simulink model "sampleModel1754"  (R2023a)
settings: Solver=VariableStepAuto  StartTime=0.0  StopTime=10.0  RelTol=1e-3
libraries: hdlsllib x5, simulink x1
settings Model: Creator=user1  LastModifiedBy=user1

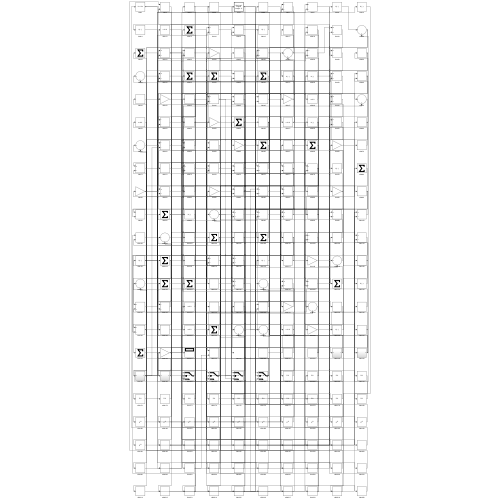
[thumbnail: Simulink's stored preview of the top-level diagram]
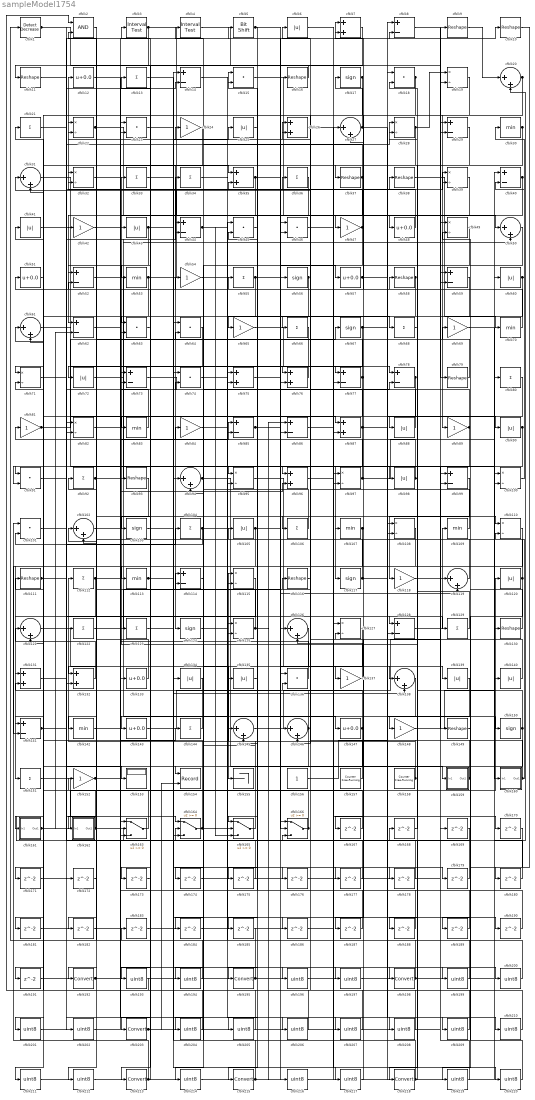
== system sampleModel1754 ==
  cfblk1 : simulink/Logic and Bit Operations/Detect Decrease  vinit=0.0  OutDataTypeStr=boolean
      settings: LibrarySourceBlock=|
      | hdlsllib/Logic and Bit
      | Operations/Detect
      | Decrease
  cfblk{9..11,16,37..38,58,79,93,111,116,130,149} (13 alike) : Reshape
  cfblk{19,22,28,32,39,49,71,82,95,97,100,108,110,115,125,127} (16 alike) : Product  Inputs=*/  RndMeth=Zero  SaturateOnIntegerOverflow=on
  cfblk{15,18,23,45..46,63..64,74,91,101,136} (11 alike) : DotProduct  OutDataTypeStr=Inherit: Inherit via internal rule
  cfblk{20,27,31,50,61,94,102,119,121,126,138,145..146} (13 alike) : Sum  Inputs=|++
  cfblk{17,56,67,103,117,124,150} (7 alike) : Signum
  cfblk{13,21,33..34,36,55,66,68,80,92,104,106,112,122..123,129,144,151} (18 alike) : Sum  Inputs=+
  cfblk{6,25,41,43,60,72,88,90,98,105,120,134..135,139..140} (15 alike) : Abs  SaturateOnIntegerOverflow=off
  cfblk{30,53,70,83,107,109,113,142} (8 alike) : MinMax
  cfblk{8,14,29,40,44,52,59,62,73,77..78,85..86,99,114,128,141} (17 alike) : Sum  Inputs=+-
  cfblk{24,42,47,54,65,69,81,84,89,118,137,148,152} (13 alike) : Gain
  cfblk{12,48,51,57,133,143,147} (7 alike) : Bias  Bias=0.0  SaturateOnIntegerOverflow=off
  cfblk{7,26,35,75..76,87,96,131..132} (9 alike) : Sum
  cfblk153 : Display
  cfblk154 : Record  FileSettingsInternal="{\"entries\":[{\"content\":{\"excelSettings\":{\"content\":{},\"type\":\"Streamout.ExcelSettings\"}},\"type\":\"Streamout.FileSettingStorage\",\"uuid\":\"\"}],\"packageUris\":[\"http:\\/\\/schema.mathworks.com\\/mf0\\/streamout_blocks\\/R2020a\"],\"version\":\"1.0\"}"  Layout=[1 1]  SignalsInternal="{\"entries\":[{\"content\":{\"signals\":[{\"content\":{\"blockPath\":[],\"dimensions\":[1],\"domain\":\"\",\"lineColor\":\"#a2142f\",\"plots\":[1],\"port\":1,\"sid\":[\"\"],\"signalID\":3756,\"signalName\":\"cfblk50\"},\"type\":\"RecordBlkView.Signal\",\"uuid\":\"\"},{\"content\":{\"blockPath\":[],\"dimensions\":[1],\"domain\":\"\",\"lineColor\":\"#139fff\",\"plots\":[1],\"port\":2,\"sid\":[\"\"],\"signalID\":3760,\"signalName\":\"cfblk203\"},\"type\":\"RecordBlkView.Signal\",\"uuid\":\"\"}]},\"type\":\"RecordBlkView.InputSignals\",\"uuid\":\"\"}],\"packageUris\":[\"http:\\/\\/schema.mathworks.com\\/mf0\\/streamout_blocks\\/R2020a\"],\"version\":\"1.0\"}"  VisualizationBindings="{\"xyplotplugin\":{\"info\":[{\"series\":[{\"bindingParametersList\":[{\"parameter\":\"X-Axis\",\"signalID\":3756,\"signalName\":\"cfblk50\"},{\"parameter\":\"Y-Axis\",\"signalID\":3760,\"signalName\":\"cfblk203\"}],\"seriesID\":56446}],\"subplotID\":1}]}}"  CompatibilityTag=XY  st=-1
  cfblk155 : Terminator
  cfblk156 : Constant  SampleTime=-1
  cfblk157 : hdlsllib/Sources/Counter Free-Running  NumBits=16  tsamp=-1
  cfblk158 : hdlsllib/Sources/Counter Free-Running  NumBits=16  tsamp=-1
  cfblk159 : Subsystem
      settings: LibrarySourceBlock=|
      | hdlsllib/Ports &
      | Subsystems/Subsystem
  cfblk160 : Subsystem
      settings: LibrarySourceBlock=|
      | hdlsllib/Ports &
      | Subsystems/Subsystem
  cfblk161 : Subsystem
      settings: LibrarySourceBlock=|
      | hdlsllib/Ports &
      | Subsystems/Subsystem
  cfblk162 : Subsystem
      settings: LibrarySourceBlock=|
      | hdlsllib/Ports &
      | Subsystems/Subsystem
  cfblk{163..166} (4 alike) : Switch  SaturateOnIntegerOverflow=off  InputSameDT=off
  cfblk{167..191} (25 alike) : Delay  SampleTime=1
  cfblk{192,195,198,203,213,215,218} (7 alike) : DataTypeConversion  SaturateOnIntegerOverflow=off  RndMeth=Floor
  cfblk{193..194,196..197,199..202,204..212,214,216..217,219..220} (22 alike) : DataTypeConversion  OutDataTypeStr=uint8  SaturateOnIntegerOverflow=off  RndMeth=Floor
  cfblk2 : Logic  AllPortsSameDT=off  OutDataTypeStr=boolean
  cfblk3 : hdlsllib/Logic and Bit Operations/Interval Test  IntervalClosedRight=on  uplimit=0.5  IntervalClosedLeft=on  lowlimit=-0.5  OutDataTypeStr=boolean
  cfblk4 : hdlsllib/Logic and Bit Operations/Interval Test  IntervalClosedRight=on  uplimit=0.5  IntervalClosedLeft=on  lowlimit=-0.5  OutDataTypeStr=boolean
  cfblk5 : hdlsllib/Logic and Bit Operations/Bit Shift  mode=Shift Left Logical  N=0
  wires:
  cfblk139/1 -> cfblk143/1
  cfblk158/1 -> cfblk112/1, cfblk123/1
  cfblk110/1 -> cfblk151/1
  cfblk22/1 -> cfblk50/1, cfblk35/1
  cfblk41/1 -> cfblk78/1
  cfblk125/1 -> cfblk102/1, cfblk146/1
  cfblk161/1(Out1) -> cfblk120/1, cfblk62/2, cfblk5/1, cfblk39/2, cfblk191/1
  cfblk52/1 -> cfblk155/1
  cfblk104/1 -> cfblk147/1, cfblk101/2
  cfblk85/1 -> cfblk86/1, cfblk138/1, cfblk216/1
  cfblk93/1 -> cfblk132/1
  cfblk95/1 -> cfblk137/1
  cfblk147/1 -> cfblk71/2, cfblk193/1
  cfblk92/1 -> cfblk50/2, cfblk106/1
  cfblk136/1 -> cfblk33/1
  cfblk9/1 -> cfblk20/1
  cfblk87/1 -> cfblk95/1, cfblk39/1, cfblk103/1, cfblk54/1
  cfblk119/1 -> cfblk43/1
  cfblk59/1 -> cfblk195/1
  cfblk156/1 -> cfblk8/1
  cfblk116/1 -> cfblk6/1
  cfblk28/1 -> cfblk19/1, cfblk128/2
  cfblk133/1 -> cfblk92/1
  cfblk94/1 -> cfblk159/1(In1), cfblk165/3
  cfblk129/1 -> cfblk58/1
  cfblk2/1 -> cfblk192/1
  cfblk68/1 -> cfblk88/1
  cfblk78/1 -> cfblk184/1, cfblk214/1
  cfblk67/1 -> cfblk96/1, cfblk90/1
  cfblk29/1 -> cfblk124/1
  cfblk105/1 -> cfblk113/1, cfblk107/1
  cfblk19/1 -> cfblk89/1
  cfblk30/1 -> cfblk37/1, cfblk98/1
  cfblk15/1 -> cfblk48/1
  cfblk81/1 -> cfblk67/1, cfblk28/1
  cfblk18/1 -> cfblk163/3, cfblk167/1
  cfblk166/1 -> cfblk115/1, cfblk22/2
  cfblk31/1 -> cfblk86/2
  cfblk99/1 -> cfblk118/1
  cfblk112/1 -> cfblk131/1, cfblk85/1
  cfblk3/1 -> cfblk47/1, cfblk182/1
  cfblk141/1 -> cfblk20/2, cfblk44/2
  cfblk88/1 -> cfblk15/1
  cfblk159/1(Out1) -> cfblk114/1, cfblk28/2
  cfblk61/1 -> cfblk130/1
  cfblk121/1 -> cfblk145/1
  cfblk124/1 -> cfblk75/2
  cfblk38/1 -> cfblk70/1
  cfblk132/1 -> cfblk121/1
  cfblk82/1 -> cfblk34/1
  cfblk33/1 -> cfblk134/1
  cfblk122/1 -> cfblk56/1
  cfblk109/1 -> cfblk36/1
  cfblk97/1 -> cfblk60/1, cfblk61/2
  cfblk148/1 -> cfblk140/1
  cfblk144/1 -> cfblk41/1
  cfblk60/1 -> cfblk30/1, cfblk161/1(In1)
  cfblk25/1 -> cfblk165/1
  cfblk149/1 -> cfblk69/1
  cfblk53/1 -> cfblk38/1, cfblk71/1, cfblk186/1
  cfblk123/1 -> cfblk25/1
  cfblk127/1 -> cfblk215/1
  cfblk138/1 -> cfblk148/1
  cfblk37/1 -> cfblk53/1, cfblk4/1, cfblk187/1
  cfblk56/1 -> cfblk145/2, cfblk173/1
  cfblk89/1 -> cfblk55/1, cfblk91/2
  cfblk51/1 -> cfblk141/1
  cfblk48/1 -> cfblk12/1
  cfblk100/1 -> cfblk40/2
  cfblk164/1 -> cfblk31/2, cfblk177/1, cfblk178/1
  cfblk130/1 -> cfblk51/1
  cfblk1/1 -> cfblk29/2, cfblk164/3
  cfblk55/1 -> cfblk8/2, cfblk82/2
  cfblk76/1 -> cfblk72/1
  cfblk66/1 -> cfblk162/1(In1)
  cfblk71/1 -> cfblk153/1
  cfblk50/1 -> cfblk154/1
  cfblk34/1 -> cfblk125/1
  cfblk108/1 -> cfblk141/2
  cfblk107/1 -> cfblk132/2, cfblk194/1
  cfblk128/1 -> cfblk109/1
  cfblk8/1 -> cfblk79/1
  cfblk165/1 -> cfblk114/2
  cfblk11/1 -> cfblk122/1
  cfblk120/1 -> cfblk105/1, cfblk189/1
  cfblk131/1 -> cfblk10/1
  cfblk45/1 -> cfblk65/1
  cfblk101/1 -> cfblk128/1
  cfblk117/1 -> cfblk150/1, cfblk32/2
  cfblk151/1 -> cfblk164/1
  cfblk90/1 -> cfblk117/1, cfblk166/2
  cfblk146/1 -> cfblk24/1, cfblk211/1
  cfblk44/1 -> cfblk87/1, cfblk165/2
  cfblk163/1 -> cfblk152/1
  cfblk134/1 -> cfblk131/2
  cfblk79/1 -> cfblk26/1
  cfblk16/1 -> cfblk11/1
  cfblk113/1 -> cfblk190/1, cfblk217/1
  cfblk4/1 -> cfblk126/1
  cfblk65/1 -> cfblk77/1
  cfblk111/1 -> cfblk14/2, cfblk104/1, cfblk74/2
  cfblk98/1 -> cfblk35/2, cfblk188/1
  cfblk47/1 -> cfblk26/2, cfblk85/2
  cfblk150/1 -> cfblk125/2, cfblk212/1
  cfblk137/1 -> cfblk126/2
  cfblk43/1 -> cfblk62/1, cfblk142/1, cfblk138/2
  cfblk20/1 -> cfblk91/1, cfblk171/1
  cfblk143/1 -> cfblk16/1
  cfblk13/1 -> cfblk198/1
  cfblk49/1 -> cfblk218/1
  cfblk118/1 -> cfblk119/1
  cfblk160/1(Out1) -> cfblk22/1, cfblk135/1, cfblk110/2
  cfblk75/1 -> cfblk166/1
  cfblk35/1 -> cfblk99/2, cfblk73/2
  cfblk142/1 -> cfblk7/1
  cfblk83/1 -> cfblk73/1
  cfblk42/1 -> cfblk87/2
  cfblk27/1 -> cfblk17/1, cfblk209/1
  cfblk77/1 -> cfblk121/2, cfblk97/2, cfblk52/2
  cfblk62/1 -> cfblk93/1
  cfblk72/1 -> cfblk149/1
  cfblk106/1 -> cfblk32/1
  cfblk54/1 -> cfblk110/1
  cfblk73/1 -> cfblk78/2
  cfblk5/1 -> cfblk119/2, cfblk57/1, cfblk205/1
  cfblk162/1(Out1) -> cfblk61/1, cfblk164/2
  cfblk40/1 -> cfblk52/1, cfblk146/2
  cfblk14/1 -> cfblk68/1
  cfblk80/1 -> cfblk213/1
  cfblk57/1 -> cfblk129/1, cfblk7/2
  cfblk17/1 -> cfblk76/1, cfblk66/1
  cfblk145/1 -> cfblk9/1
  cfblk86/1 -> cfblk139/1
  cfblk140/1 -> cfblk31/1
  cfblk157/1 -> cfblk81/1
  cfblk70/1 -> cfblk27/2
  cfblk152/1 -> cfblk96/2, cfblk144/1
  cfblk58/1 -> cfblk83/1, cfblk95/2
  cfblk63/1 -> cfblk3/1
  cfblk64/1 -> cfblk203/1
  cfblk69/1 -> cfblk160/1(In1)
  cfblk7/1 -> cfblk63/1
  cfblk36/1 -> cfblk42/1
  cfblk32/1 -> cfblk44/1
  cfblk167/1 -> cfblk75/1
  cfblk168/1 -> cfblk18/2
  cfblk169/1 -> cfblk166/3
  cfblk26/1 -> cfblk170/1
  cfblk91/1 -> cfblk172/1
  cfblk172/1 -> cfblk102/2
  cfblk173/1 -> cfblk63/2
  cfblk126/1 -> cfblk174/1
  cfblk174/1 -> cfblk27/1
  cfblk39/1 -> cfblk175/1
  cfblk175/1 -> cfblk163/1
  cfblk103/1 -> cfblk176/1
  cfblk176/1 -> cfblk99/1
  cfblk177/1 -> cfblk14/1
  cfblk178/1 -> cfblk82/1
  cfblk6/1 -> cfblk179/1
  cfblk179/1 -> cfblk29/1
  cfblk10/1 -> cfblk180/1
  cfblk180/1 -> cfblk100/1
  cfblk24/1 -> cfblk181/1
  cfblk181/1 -> cfblk97/1
  cfblk183/1 -> cfblk94/1
  cfblk184/1 -> cfblk76/2
  cfblk135/1 -> cfblk185/1
  cfblk185/1 -> cfblk1/1
  cfblk186/1 -> cfblk77/2
  cfblk187/1 -> cfblk163/2
  cfblk188/1 -> cfblk15/2
  cfblk189/1 -> cfblk45/2
  cfblk190/1 -> cfblk115/2
  cfblk191/1 -> cfblk19/2
  cfblk192/1 -> cfblk133/1, cfblk40/1
  cfblk193/1 -> cfblk2/1
  cfblk194/1 -> cfblk2/2
  cfblk195/1 -> cfblk108/2, cfblk45/1
  cfblk12/1 -> cfblk196/1
  cfblk196/1 -> cfblk59/1
  cfblk182/1 -> cfblk197/1
  cfblk197/1 -> cfblk59/2
  cfblk198/1 -> cfblk100/2, cfblk116/1
  cfblk74/1 -> cfblk199/1
  cfblk199/1 -> cfblk13/1
  cfblk23/1 -> cfblk200/1
  cfblk200/1 -> cfblk18/1
  cfblk115/1 -> cfblk201/1
  cfblk201/1 -> cfblk23/1
  cfblk171/1 -> cfblk202/1
  cfblk202/1 -> cfblk23/2
  cfblk203/1 -> cfblk169/1, cfblk154/2
  cfblk114/1 -> cfblk204/1
  cfblk204/1 -> cfblk64/1
  cfblk205/1 -> cfblk64/2
  cfblk21/1 -> cfblk206/1
  cfblk206/1 -> cfblk111/1
  cfblk102/1 -> cfblk207/1
  cfblk207/1 -> cfblk21/1
  cfblk84/1 -> cfblk208/1
  cfblk208/1 -> cfblk136/2
  cfblk209/1 -> cfblk84/1
  cfblk46/1 -> cfblk210/1
  cfblk210/1 -> cfblk136/1
  cfblk211/1 -> cfblk46/1
  cfblk212/1 -> cfblk46/2
  cfblk213/1 -> cfblk183/1, cfblk101/1
  cfblk214/1 -> cfblk80/1
  cfblk215/1 -> cfblk74/1, cfblk108/1
  cfblk216/1 -> cfblk127/1
  cfblk217/1 -> cfblk127/2
  cfblk218/1 -> cfblk168/1, cfblk94/2
  cfblk170/1 -> cfblk219/1
  cfblk219/1 -> cfblk49/1
  cfblk96/1 -> cfblk220/1
  cfblk220/1 -> cfblk49/2

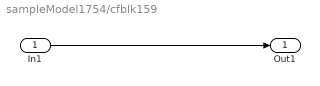
== system sampleModel1754/cfblk159 ==
  In1 : Inport
  Out1 : Outport
  wires:
  In1/1 -> Out1/1

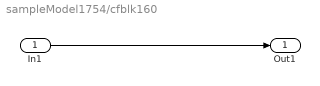
== system sampleModel1754/cfblk160 ==
  In1 : Inport
  Out1 : Outport
  wires:
  In1/1 -> Out1/1

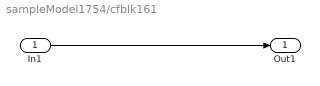
== system sampleModel1754/cfblk161 ==
  In1 : Inport
  Out1 : Outport
  wires:
  In1/1 -> Out1/1

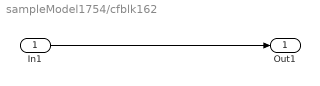
== system sampleModel1754/cfblk162 ==
  In1 : Inport
  Out1 : Outport
  wires:
  In1/1 -> Out1/1
